simulink model "sim_LQ_nonlinear"  (R2017b)
settings: Solver=VariableStepAuto  StartTime=0.0  StopTime=50  RelTol=1e-3
values from neighbouring files (symbols this model uses):
  g = 9.81    [init_sim.m]
  m = 0.03    [init_sim.m]
  Ts = 1e-2    (= 0.01)    [init_sim.m]
  x0 = zeros(6,1)    [get_sim_data.m]    (also in get_sim_data_mpc_phi.m; get_sim_data_mpc_y.m; get_sim_data_mpc_z.m; init_sim.m = 0.9*[InvSet_y.V(i,1)'; InvSet_z.V(j,1)'; InvSet_phi.V(k,1)';)
undefined symbols (not defined in the file or in its folder): K_phi1, K_phi3, K_y, K_z, uavPlanarNonlin
settings Model: Creator=zboucek  LastModifiedBy=zboucek

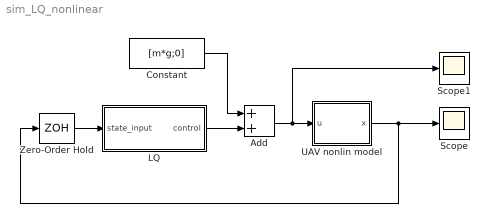
== system sim_LQ_nonlinear ==
  Add : Sum
  Constant : Constant  Value=[m*g;0]  VectorParams1D=off
  LQ : Subsystem
  Scope : Scope
  Scope1 : Scope
  UAV nonlin model : Subsystem
  Zero-Order Hold : ZeroOrderHold  SampleTime=Ts
  wires:
  UAV nonlin model/1(x) -> Zero-Order Hold/1, Scope/1
  Zero-Order Hold/1 -> LQ/1(state_input)
  LQ/1(control) -> Add/2
  Add/1 -> UAV nonlin model/1(u), Scope1/1
  Constant/1 -> Add/1

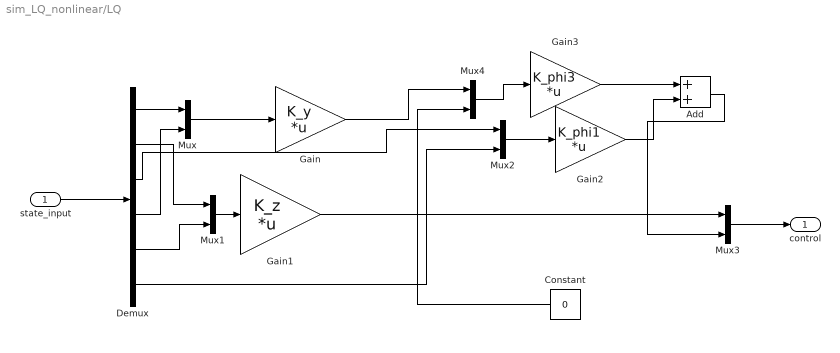
== system sim_LQ_nonlinear/LQ ==
  state_input : Inport
  Add : Sum
  Constant : Constant  Value=0
  Demux : Demux  Outputs=6
  Gain : Gain  Gain=K_y  Multiplication=Matrix(K*u) (u vector)
  Gain1 : Gain  Gain=K_z  Multiplication=Matrix(K*u) (u vector)
  Gain2 : Gain  Gain=K_phi1  Multiplication=Matrix(K*u) (u vector)
  Gain3 : Gain  Gain=K_phi3  Multiplication=Matrix(K*u) (u vector)
  Mux{,1..4} (5 alike) : Mux  Inputs=2
  control : Outport
  wires:
  state_input/1 -> Demux/1
  Demux/1 -> Mux/1
  Demux/4 -> Mux/2
  Demux/5 -> Mux1/2
  Demux/2 -> Mux1/1
  Demux/6 -> Mux2/2
  Mux/1 -> Gain/1
  Mux1/1 -> Gain1/1
  Mux3/1 -> control/1
  Gain1/1 -> Mux3/1
  Demux/3 -> Mux2/1
  Mux2/1 -> Gain2/1
  Gain2/1 -> Add/2
  Mux4/1 -> Gain3/1
  Gain/1 -> Mux4/1
  Gain3/1 -> Add/1
  Add/1 -> Mux3/2
  Constant/1 -> Mux4/2

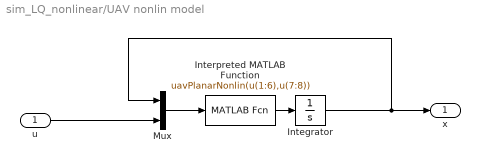
== system sim_LQ_nonlinear/UAV nonlin model ==
  u : Inport
  Integrator : Integrator  InitialCondition=x0
  Interpreted MATLAB Function : MATLABFcn  MATLABFcn=uavPlanarNonlin(u(1:6),u(7:8))  OutputDimensions=6
  Mux : Mux  Inputs=2
  x : Outport
  wires:
  Mux/1 -> Interpreted MATLAB Function/1
  Interpreted MATLAB Function/1 -> Integrator/1
  Integrator/1 -> x/1, Mux/1
  u/1 -> Mux/2
